simulink model "sphere_position_model"  (R2021a)
settings: Solver=FixedStepAuto  StartTime=0.0  StopTime=10.0  FixedStep=0.1  RelTol=1e-3
settings Model: Creator=dupa1607  LastModifiedBy=antho
settings SolverCC: AlgebraicLoopSolver=TrustRegion
settings DebuggingCC: SFMachineParentedDataDiag=warning

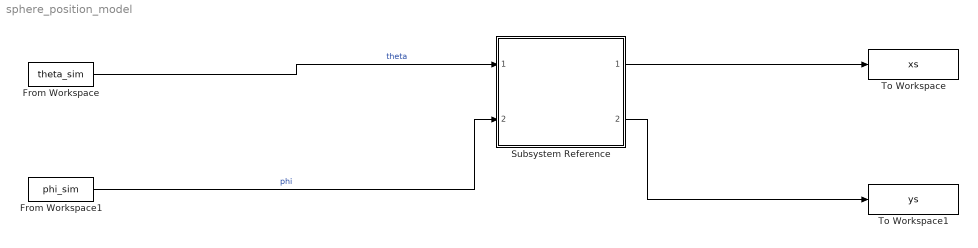
== system sphere_position_model ==
  From Workspace : FromWorkspace  VariableName=theta_sim
  From Workspace1 : FromWorkspace  VariableName=phi_sim
  Subsystem Reference : Subsystem  ReferencedSubsystem=subsys_sphere_position
  To Workspace : ToWorkspace  VariableName=xs  SaveFormat=Timeseries  SampleTime=-1
  To Workspace1 : ToWorkspace  VariableName=ys  SaveFormat=Timeseries  SampleTime=-1
  wires:
  From Workspace/1 -> Subsystem Reference/1  "theta"
  From Workspace1/1 -> Subsystem Reference/2  "phi"
  Subsystem Reference/1 -> To Workspace/1
  Subsystem Reference/2 -> To Workspace1/1
